simulink model "Lab 1_1 and 2"  (R2026a)
settings: Solver=VariableStepAuto  StopTime=inf
undefined symbols (not defined in the file): Blocking, Non
libraries: fl_lib x9, nesl_utility x6, ee_lib x2, amg_usbconverter_n_connect_lib x2
settings Model: Creator=Asus  LastModifiedBy=Asus

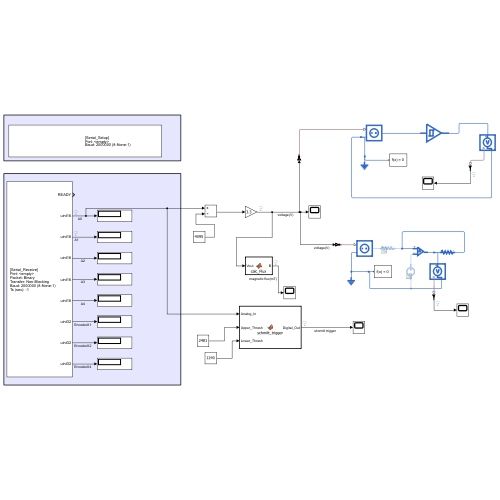
[thumbnail: Simulink's stored preview of the top-level diagram]
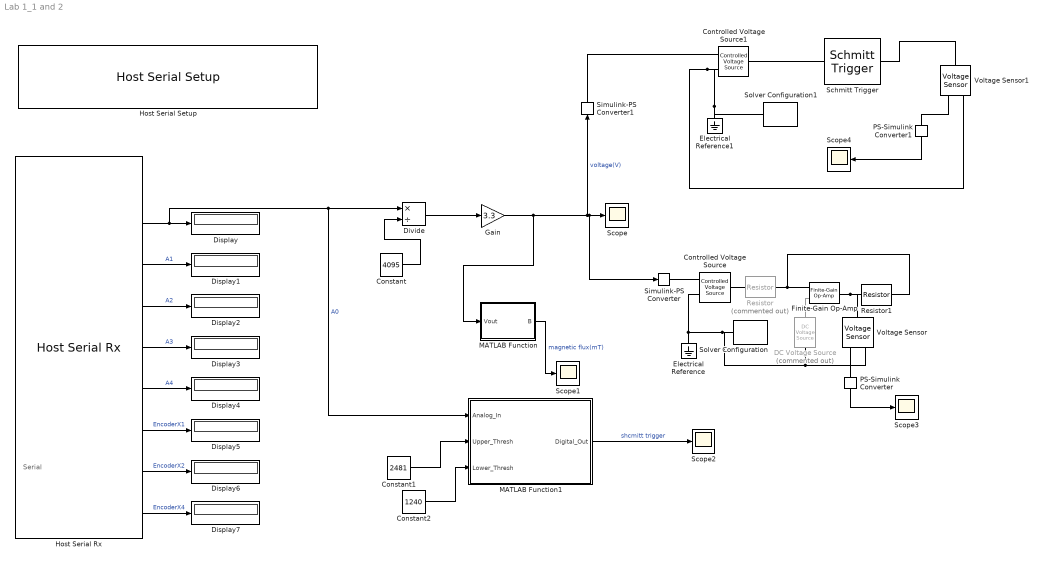
== system Lab 1_1 and 2 ==
  note: Serial
  Constant : Constant  Value=4095
  Constant1 : Constant  Value=2481
  Constant2 : Constant  Value=1240
  Controlled Voltage Source : fl_lib/Electrical/Electrical Sources/Controlled Voltage Source
  Controlled Voltage Source1 : fl_lib/Electrical/Electrical Sources/Controlled Voltage Source
  DC Voltage Source : fl_lib/Electrical/Electrical Sources/DC Voltage Source  Commented=on  v0=1.535 V
  Display{,1..7} (8 alike) : Display
  Divide : Product  Inputs=*/
  Electrical Reference : fl_lib/Electrical/Electrical Elements/Electrical Reference
  Electrical Reference1 : fl_lib/Electrical/Electrical Elements/Electrical Reference
  Finite-Gain Op-Amp : ee_lib/Integrated Circuits/Finite-Gain Op-Amp  A=1000  Rin=1e6 Ohm  Rout=100 Ohm  Vmin=0 V  Vmax=1 V  noise_mode=ee.enum.mode.disabled  v_noise=30e-9 V/Hz^(1/2)  noise_prm=ee.enum.ic.noiseParameterization.same  i_noise=0.5e-12 A/Hz^(1/2)  ip_noise=0.5e-12 A/Hz^(1/2)  in_noise=0.5e-12 A/Hz^(1/2)  sample_time=1e-3 s  repeatability=ee.enum.ic.repeatability.notRepeatable  auto_seed_v=3922919431  auto_seed_ip=2715962282  auto_seed_in=418932850  user_seed_v=0  user_seed_ip=0  user_seed_in=0
  Gain : Gain  Gain=3.3
  Host Serial Rx : amg_usbconverter_n_connect_lib/Host Serial Rx  conf=rx  port=<auto>  baudrate=2000000  databits=8  parity=None  stopbit=1  flowcontrol=None  transfer=Non-Blocking  timeout=5  packetmode=Binary  enableinitialvalues=off  initialvalues=[]  binheader='25'  binterminator='4E 4E'  porttype_double=0  porttype_single=0  porttype_int8=0  porttype_uint8=0  porttype_int16=0  porttype_uint16=5  porttype_int32=0  porttype_uint32=3  asciiformat='%d,%f'  rx_asciiterminator="CRLF (0x0D 0x0A - \"\\r\\n\")"  tx_asciiterminator="CRLF (0x0D 0x0A - \"\\r\\n\")"  sampletime=0.001  enablecustomportlabel=off  cinputportlabel=0  coutputportlabel=A  portpinstr=0  blockid=HostSerialRx  inputporttype=[]  inputportwidth=[]  inputportlabel={}  outputporttype=[3 5 5 5 5 5 7 7 7]  outputportwidth=[1 1 1 1 1 1 1 1 1]  outputportlabel={'READY','uint16','uint16','uint16','uint16','uint16','uint32','uint32','uint32'}  compat=0  optionstring=[]  autoport='<empty>'
  Host Serial Setup : amg_usbconverter_n_connect_lib/Host Serial Setup  conf=setup  port=<auto>  baudrate=2000000  databits=8  parity=None  stopbit=1  flowcontrol=None  transfer=Blocking  timeout=2  packetmode=Binary  initialvalues=[]  binheader='7E 7E'  binterminator='03 03'  porttype_double=0  porttype_single=1  porttype_int8=0  porttype_uint8=0  porttype_int16=0  porttype_uint16=0  porttype_int32=0  porttype_uint32=2  asciiformat='%d %u %x'  rx_asciiterminator="CRLF (0x0D 0x0A - \"\\r\\n\")"  tx_asciiterminator="CRLF (0x0D 0x0A - \"\\r\\n\")"  sampletime=-1  enablecustomportlabel=off  cinputportlabel=0  coutputportlabel=A  portpinstr=0  blockid=HostSerialSetup  inputporttype=[]  inputportwidth=[]  inputportlabel={}  outputporttype=[]  outputportwidth=[]  outputportlabel={}  compat=0  optionstring=[]  autoport='<empty>'
  MATLAB Function : MATLAB Function  TreatAsAtomicUnit=on
  MATLAB Function1 : MATLAB Function  TreatAsAtomicUnit=on
  PS-Simulink Converter : nesl_utility/PS-Simulink Converter  PhysicalDomain=network_engine_domain  SubClassName=ps_output  LeftPortType=input  RightPortType=output  PseudoPeriodic=off  Frequencies=[]  VectorFormat=inherit  Unit=inherit  AffineConversion=off
  PS-Simulink Converter1 : nesl_utility/PS-Simulink Converter  PhysicalDomain=network_engine_domain  SubClassName=ps_output  LeftPortType=input  RightPortType=output  PseudoPeriodic=off  Frequencies=[]  VectorFormat=inherit  Unit=inherit  AffineConversion=off
  Resistor : fl_lib/Electrical/Electrical Elements/Resistor  Commented=on  R=10 kOhm  i_specify=off  i_priority=None  i=0 A  i_nominal_specify=off  i_nominal_value=1  i_nominal_unit=A  v_specify=off  v_priority=None  v=0 V  v_nominal_specify=off  v_nominal_value=1  v_nominal_unit=V
  Resistor1 : fl_lib/Electrical/Electrical Elements/Resistor  R=33 kOhm  i_specify=off  i_priority=None  i=0 A  i_nominal_specify=off  i_nominal_value=1  i_nominal_unit=A  v_specify=off  v_priority=None  v=0 V  v_nominal_specify=off  v_nominal_value=1  v_nominal_unit=V
  Schmitt Trigger : ee_lib/Integrated Circuits/Logic/Schmitt Trigger  V_IL=1 V  V_IH=2 V  C_IN=5 pF  output_type=ee.enum.ic.outputType.linear  V_OL=0 V  V_OH=1 V  V_CC=5 V  V_meas=5 V  R_OUT=25 Ohm  R_OH=[25, 250] Ohm  I_OH=63 mA  R_OL=[30, 800] Ohm  I_OL=-45 mA  Delay=25 ns  Ron=5 Ohm  Vf=0.6 V  output_state=ee.enum.ic.initialState.low
  Scope{,1..4} (5 alike) : Scope
      Scope settings: ActiveDisplayYMinimum=-29.471685212947058  ActiveDisplayYMaximum=19.265337201699708
      Scope2 settings: DataLoggingVariableName=ScopeData2
      Scope3 settings: DataLoggingVariableName=ScopeData3
      Scope4 settings: DataLoggingVariableName=ScopeData4
  Simulink-PS Converter : nesl_utility/Simulink-PS Converter  PhysicalDomain=network_engine_domain  SubClassName=ps_input  LeftPortType=input  RightPortType=output  PseudoPeriodic=off  Frequencies=[]  NoiseDistribution=none  NoiseParameters=[]  Unit=V  AffineConversion=off  FilteringAndDerivatives=filter  SimscapeFilterOrder=1  InputFilterTimeConstant=0.001  UdotUserProvided=0
  Simulink-PS Converter1 : nesl_utility/Simulink-PS Converter  PhysicalDomain=network_engine_domain  SubClassName=ps_input  LeftPortType=input  RightPortType=output  PseudoPeriodic=off  Frequencies=[]  NoiseDistribution=none  NoiseParameters=[]  Unit=V  AffineConversion=off  FilteringAndDerivatives=filter  SimscapeFilterOrder=1  InputFilterTimeConstant=0.001  UdotUserProvided=0
  Solver Configuration : nesl_utility/Solver Configuration  PhysicalDomain=network_engine_domain  SubClassName=solver  LeftPortType=input  RightPortType=generic  Tones=[]  Harmonics=[]  SimulateNoise=off  Profile=off  UseLocalSampling=off  EnableSwitchedLinearOptims=on  FrequencyDomain=off  UseCCode=off  RelTol=0.001  AbsTol=0.001  MinStep=1e-09  ToWorkspace=off  RevertToSquareIcSolve=off  NumHomotopyIterations=100  PhasorMode=off  PhasorModeNumHarmonics=1  ConsistencySolver=NEWTON_XTOL_AFTER_FTOL  CanonicalOrdering=CANONICAL  OptimizeIntermediates=OPTIMIZED  IndexReductionMethod=DerivativeReplacement  DoDC=off  ResidualTolerance=1e-09  ConsistencyTolSource=GLOBAL  ConsistencyAbsTol=0.001  ConsistencyRelTol=0.001  ConsistencyTolFactor=0.001  UseLocalSolver=on  LocalSolverChoice=NE_BACKWARD_EULER_ADVANCER  ResolveIndetEquations=on  FunctionEvalNumThread=1  LocalSolverSampleTime=0.001  DoFixedCost=off  MaxNonlinIter=3  MaxModeIter=2  ComputeImpulses=off  ImpulseIterations=2  LinearAlgebra=auto  LinearAlgebraNumThread=0  EquationFormulation=NE_TIME_EF  DelaysMemoryBudget=1024  AutomaticFiltering=on  FilteringTimeConstant=0.001  PartitionStorageMethod=AS_NEEDED  PartitionMemoryBudget=1024  PartitionMethod=ROBUST  MultibodyUseLocalSolver=off  MultibodyLocalSolverChoice=ODE1  MultibodyLocalSolverSampleTime=0.001
  Solver Configuration1 : nesl_utility/Solver Configuration  PhysicalDomain=network_engine_domain  SubClassName=solver  LeftPortType=input  RightPortType=generic  Tones=[]  Harmonics=[]  SimulateNoise=off  Profile=off  UseLocalSampling=off  EnableSwitchedLinearOptims=on  FrequencyDomain=off  UseCCode=off  RelTol=0.001  AbsTol=0.001  MinStep=1e-09  ToWorkspace=off  RevertToSquareIcSolve=off  NumHomotopyIterations=100  PhasorMode=off  PhasorModeNumHarmonics=1  ConsistencySolver=NEWTON_XTOL_AFTER_FTOL  CanonicalOrdering=CANONICAL  OptimizeIntermediates=OPTIMIZED  IndexReductionMethod=DerivativeReplacement  DoDC=off  ResidualTolerance=1e-09  ConsistencyTolSource=GLOBAL  ConsistencyAbsTol=0.001  ConsistencyRelTol=0.001  ConsistencyTolFactor=0.001  UseLocalSolver=on  LocalSolverChoice=NE_BACKWARD_EULER_ADVANCER  ResolveIndetEquations=on  FunctionEvalNumThread=1  LocalSolverSampleTime=0.001  DoFixedCost=off  MaxNonlinIter=3  MaxModeIter=2  ComputeImpulses=off  ImpulseIterations=2  LinearAlgebra=auto  LinearAlgebraNumThread=0  EquationFormulation=NE_TIME_EF  DelaysMemoryBudget=1024  AutomaticFiltering=on  FilteringTimeConstant=0.001  PartitionStorageMethod=AS_NEEDED  PartitionMemoryBudget=1024  PartitionMethod=ROBUST  MultibodyUseLocalSolver=off  MultibodyLocalSolverChoice=ODE1  MultibodyLocalSolverSampleTime=0.001
  Voltage Sensor : fl_lib/Electrical/Electrical Sensors/Voltage Sensor
  Voltage Sensor1 : fl_lib/Electrical/Electrical Sensors/Voltage Sensor
  wires:
  PS-Simulink Converter/1 -> Scope3/1
  Host Serial Rx/5 -> Display3/1  "A3"
  Host Serial Rx/8 -> Display6/1  "EncoderX2"
  Host Serial Rx/7 -> Display5/1  "EncoderX1"
  Constant2/1 -> MATLAB Function1/3(Lower_Thresh)
  PS-Simulink Converter1/1 -> Scope4/1
  MATLAB Function/1(B) -> Scope1/1  "magnetic flux(mT)"
  Divide/1 -> Gain/1
  Constant/1 -> Divide/2
  Host Serial Rx/3 -> Display1/1  "A1"
  Host Serial Rx/4 -> Display2/1  "A2"
  Host Serial Rx/9 -> Display7/1  "EncoderX4"
  Gain/1 -> MATLAB Function/1(Vout), Simulink-PS Converter1/1, Simulink-PS Converter/1, Scope/1  "voltage(V)"
  MATLAB Function1/1(Digital_Out) -> Scope2/1  "shcmitt trigger"
  Host Serial Rx/2 -> MATLAB Function1/1(Analog_In), Divide/1, Display/1  "A0"
  Constant1/1 -> MATLAB Function1/2(Upper_Thresh)
  Host Serial Rx/6 -> Display4/1  "A4"
  connections:
  Controlled Voltage Source/RConn2 -- Voltage Sensor/RConn2 -- DC Voltage Source/RConn1 -- Solver Configuration/RConn1 -- Electrical Reference/LConn1
  Voltage Sensor1/RConn2 -- Controlled Voltage Source1/RConn2 -- Solver Configuration1/RConn1 -- Electrical Reference1/LConn1
  Finite-Gain Op-Amp/RConn1 -- Voltage Sensor/LConn1 -- Resistor1/LConn1
  Finite-Gain Op-Amp/LConn1 -- Resistor1/RConn1 -- Resistor/RConn1
  Voltage Sensor1/RConn1 -- PS-Simulink Converter1/LConn1
  Controlled Voltage Source1/RConn1 -- Simulink-PS Converter1/RConn1
  Controlled Voltage Source1/LConn1 -- Schmitt Trigger/LConn1
  Controlled Voltage Source/RConn1 -- Simulink-PS Converter/RConn1
  DC Voltage Source/LConn1 -- Finite-Gain Op-Amp/LConn2
  PS-Simulink Converter/LConn1 -- Voltage Sensor/RConn1
  Controlled Voltage Source/LConn1 -- Resistor/LConn1
  Schmitt Trigger/RConn1 -- Voltage Sensor1/LConn1

== matlab function Lab 1_1 and 2/MATLAB Function ==
  data: Vout input; B output
function B = calc_Flux (Vout)
    VQ = 1650;
    Sens25 = 30;
    STC = 0.0012;
    TA = 25;

    S_TA =Sens25 * (1 + STC * (TA - 25));

    B = (Vout - VQ) / S_TA;
end

== matlab function Lab 1_1 and 2/MATLAB Function1 ==
  data: Analog_In input; Digital_Out output; Upper_Thresh input; Lower_Thresh input
function Digital_Out = schmitt_trigger(Analog_In, Upper_Thresh, Lower_Thresh)
% อธิบายโปรแกรม (ตาม Criteria ภาคผนวก):
% ฟังก์ชันนี้รับค่า Analog_In จาก Potentiometer
% และเปรียบเทียบกับค่า Upper และ Lower Threshold ที่ตั้งไว้

% กำหนดตัวแปร persistent เพื่อจดจำสถานะเอาต์พุตในรอบการทำงาน (Step) ก่อนหน้า
persistent state;

% กำหนดค่าเริ่มต้นให้กับ state เมื่อโปรแกรมเริ่มทำงานครั้งแรก
if isempty(state)
    state = 0; 
end

% ลอจิกการทำงานของ Schmitt Trigger
if Analog_In >= Upper_Thresh
    state = 1; % สัญญาณเปลี่ยนเป็น HIGH เมื่อเกินขีดจำกัดบน
elseif Analog_In <= Lower_Thresh
    state = 0; % สัญญาณเปลี่ยนเป็น LOW เมื่อต่ำกว่าขีดจำกัดล่าง
end

% ส่งค่าสถานะปัจจุบันกลับออกไปยัง Output พอร์ต
Digital_Out = state;
end
